simulink model "S_land_interfer_simulation"  (R2021a)
settings: Solver=FixedStepAuto  StartTime=0.0  StopTime=5  FixedStep=0.001  RelTol=1e-3
InitFcn:
  | Init_control;
values from neighbouring files (symbols this model uses):
  DEG2RAD = 0.0174533    [Init_control.m]
  Kd_PITCH_AgngleRate = 0.001    [Init_control.m]
  Kd_ROLL_AgngleRate = 0.001    [Init_control.m]
  Kd_YAW_AngleRate = 0.00    (= 0)    [Init_control.m]
  Ki_PITCH_AgngleRate = 0.10    (= 0.1)    [Init_control.m]
  Ki_ROLL_AgngleRate = 0.02    [Init_control.m]
  Ki_YAW_AngleRate = 0.01    [Init_control.m]
  Kp_PITCH_AgngleRate = 0.1    [Init_control.m]
  Kp_PITCH_ANGLE = 6.5    [Init_control.m]
  Kp_ROLL_AgngleRate = 0.1    [Init_control.m]
  Kp_ROLL_ANGLE = 6.5    [Init_control.m]
  Kp_YAW_AngleRate = 0.3    [Init_control.m]
  Kpxd = 0.5    [Init_control.m]
  Kpxi = 0    [Init_control.m]
  Kpxp = 5    [Init_control.m]
  Kpyp = 1.0    (= 1)    [Init_control.m]
  Kpzd = 0    [Init_control.m]
  Kpzi = 0.1    [Init_control.m]
  Kpzp = 5    [Init_control.m]
  Kvxd = 0.5    [Init_control.m]
  Kvxi = 0.01    [Init_control.m]
  Kvxp = 5    [Init_control.m]
  Kvyd = 0.01    [Init_control.m]
  Kvyi = 0    [Init_control.m]
  Kvyp = 2.0    (= 2)    [Init_control.m]
  Kvzd = 0.005    [Init_control.m]
  Kvzi = 0.01    [Init_control.m]
  Kvzp = 5    [Init_control.m]
  MAX_CONTROL_ANGLE_PITCH = 50    [Init_control.m]
  MAX_CONTROL_ANGLE_RATE_PITCH = 220    [Init_control.m]
  MAX_CONTROL_ANGLE_RATE_ROLL = 220    [Init_control.m]
  MAX_CONTROL_ANGLE_ROLL = 35    [Init_control.m]
  MAX_CONTROL_VELOCITY_XY = 5    [Init_control.m]
  MAX_CONTROL_VELOCITY_Z = 3    [Init_control.m]
  MAX_MAN_THR = 0.9    [Init_control.m]
  ModelInit_PosE = [0,0,-10]    [Init_control.m]
  ModelInit_RPM = 557.1420    (= 557.142)    [Init_control.m]
  RAD2DEG = 57.2957795    [Init_control.m]
  Saturation_I_ah = 3.431    [Init_control.m]
  Saturation_I_az = 5    [Init_control.m]
  Saturation_I_RP_Max = 0.3    [Init_control.m]
  Saturation_I_RP_Min = -0.3    [Init_control.m]
  Saturation_I_Y_Max = 0.2    [Init_control.m]
  Saturation_I_Y_Min = -0.2    [Init_control.m]
  THR_HOVER = 0.609    [Init_control.m]
undefined symbols (not defined in the file or in its folder): DiscIntNeverNeededParam, ModelParam_envGravityAcc, ModelParam_motorCr, ModelParam_motorJm, ModelParam_motorT, ModelParam_motorWb, ModelParam_rotorCm, ModelParam_rotorCt, ModelParam_uavCd, ModelParam_uavJ, ModelParam_uavMass, ModelParam_uavR
libraries: simulink x5, sharedutil x2, pid_lib x2, sharedtransform x1
settings Model: Creator=dream  LastModifiedBy=shenl
settings SolverCC: AlgebraicLoopSolver=TrustRegion
settings DataIOCC: ReturnWorkspaceOutputs=off
settings DebuggingCC: BusObjectLabelMismatch=error  SFMachineParentedDataDiag=warning  ArithmeticOperatorsInVariantConditions=warning
settings SFSimCC: SimUseLocalCustomCode=off  CustomCodeUndefinedFunction=UseInterfaceOnly
settings RTWCC: RTWUseLocalCustomCode=off
settings CodeAppCC: StateflowObjectComments=on

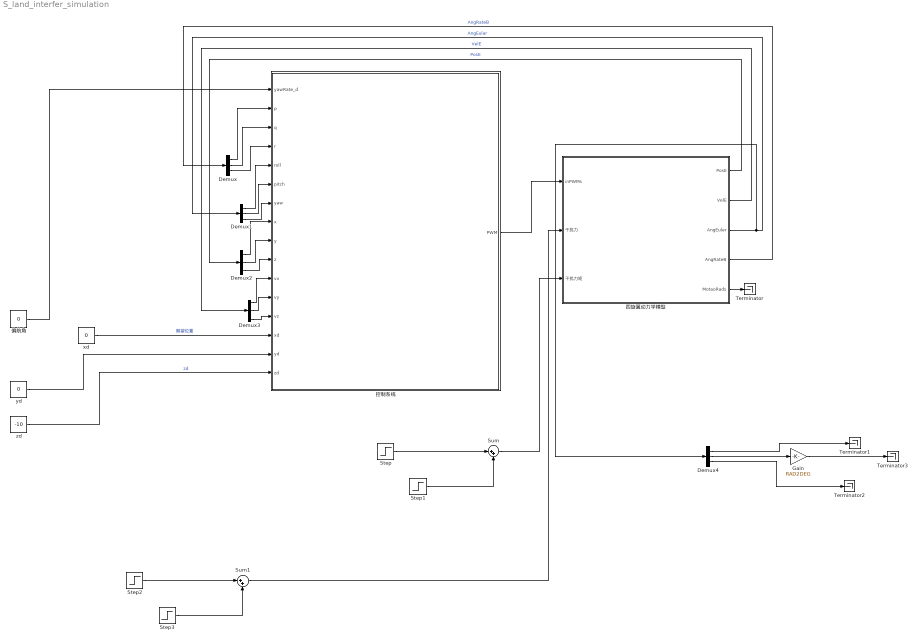
== system S_land_interfer_simulation ==
  Demux{,1..4} (5 alike) : Demux  Outputs=3
  Gain : Gain  Gain=RAD2DEG
  Step : Step  After=7  SampleTime=0
  Step1 : Step  Time=1.1  After=-6.1  SampleTime=0
  Step2 : Step  After=36  SampleTime=0
  Step3 : Step  Time=1.1  After=-30  SampleTime=0
  Sum : Sum  Inputs=|++
  Sum1 : Sum  Inputs=|++
  Terminator{,1..3} (4 alike) : Terminator
  xd : Constant  Value=0
  yd : Constant  Value=0
  zd : Constant  Value=-10
  偏航角 : Constant  Value=0  OutDataTypeStr=double
  "四旋翼动力学模型 " : Subsystem
      mask Display: image('./icon/F450.png');
  控制系统 : Subsystem
      mask Display: image('icon\pixhawk.png');
  wires:
  "四旋翼动力学模型 "/1(PosE) -> Demux2/1  "PosE"
  "四旋翼动力学模型 "/3(AngEuler) -> Demux4/1, Demux1/1  "AngEular"
  "四旋翼动力学模型 "/4(AngRateB) -> Demux/1  "AngRateB"
  Demux/1 -> 控制系统/2(p)
  Demux/2 -> 控制系统/3(q)
  Demux/3 -> 控制系统/4(r)
  Demux1/1 -> 控制系统/5(roll)
  Demux1/2 -> 控制系统/6(pitch)
  Demux1/3 -> 控制系统/7(yaw)
  Demux2/1 -> 控制系统/8(x)
  Demux2/2 -> 控制系统/9(y)
  Demux2/3 -> 控制系统/10(z)
  Demux3/1 -> 控制系统/11(vx)
  Demux3/2 -> 控制系统/12(vy)
  Demux3/3 -> 控制系统/13(vz)
  "四旋翼动力学模型 "/2(VelE) -> Demux3/1  "VelE"
  偏航角/1 -> 控制系统/1(yawRate_d)
  控制系统/1(PWM) -> "四旋翼动力学模型 "/1(inPWMs)
  "四旋翼动力学模型 "/5(MotaoRads) -> Terminator/1
  yd/1 -> 控制系统/15(yd)
  zd/1 -> 控制系统/16(zd)  "zd"
  Step/1 -> Sum/1
  Step1/1 -> Sum/2
  Sum/1 -> "四旋翼动力学模型 "/3(干扰力矩)
  Demux4/2 -> Gain/1
  Demux4/1 -> Terminator1/1
  Demux4/3 -> Terminator2/1
  Gain/1 -> Terminator3/1
  xd/1 -> 控制系统/14(xd)  "期望位置"
  Sum1/1 -> "四旋翼动力学模型 "/2(干扰力)
  Step3/1 -> Sum1/2
  Step2/1 -> Sum1/1

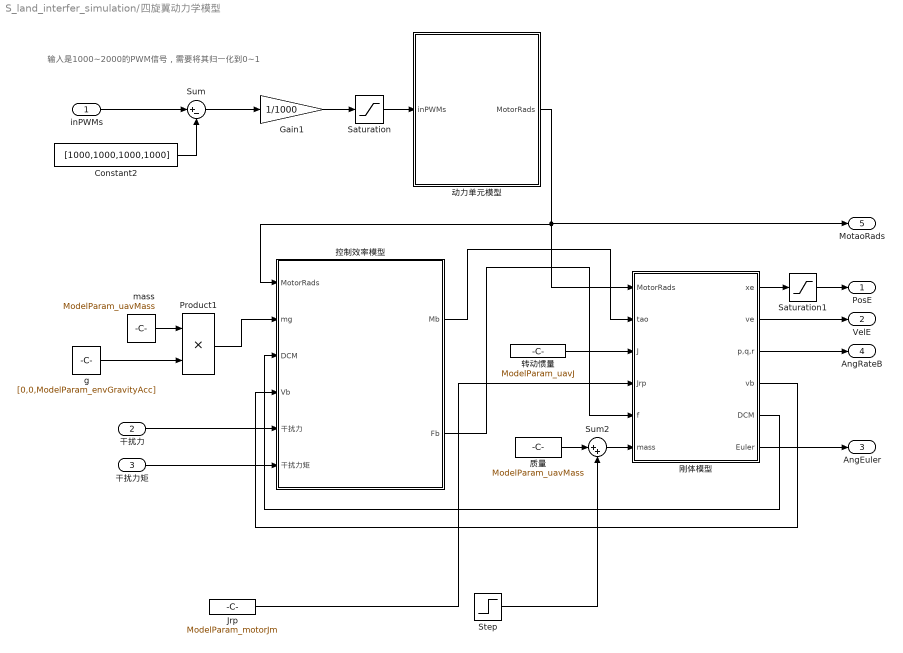
== system S_land_interfer_simulation/四旋翼动力学模型  ==
  note: 输入是1000~2000的PWM信号，需要将其归一化到0~1
  inPWMs : Inport
  干扰力 : Inport  Port=2
  干扰力矩 : Inport  Port=3
  Constant2 : Constant  Value=[1000,1000,1000,1000]
  Gain1 : Gain  Gain=1/1000
  Jrp : Constant  Value=ModelParam_motorJm
  Product1 : Product
  Saturation : Saturate  UpperLimit=1  LowerLimit=0
  Saturation1 : Saturate  UpperLimit=[inf,inf,0]  LowerLimit=[-inf,-inf,-inf]
  Step : Step  SampleTime=0
  Sum : Sum  Inputs=|+-
  Sum2 : Sum  Inputs=|++
  g : Constant  Value=[0,0,ModelParam_envGravityAcc]
  mass : Constant  Value=ModelParam_uavMass
  刚体模型 : Subsystem
  动力单元模型 : Subsystem
  控制效率模型 : Subsystem
  质量 : Constant  Value=ModelParam_uavMass
  转动惯量 : Constant  Value=ModelParam_uavJ
  PosE : Outport
  VelE : Outport  Port=2
  AngEuler : Outport  Port=3
  AngRateB : Outport  Port=4
  MotaoRads : Outport  Port=5
  wires:
  Saturation/1 -> 动力单元模型/1(inPWMs)
  刚体模型/3("p,q,r ") -> AngRateB/1
  质量/1 -> Sum2/1
  刚体模型/5(DCM) -> 控制效率模型/3(DCM)
  刚体模型/1("xe ") -> Saturation1/1
  动力单元模型/1(MotorRads) -> 控制效率模型/1(MotorRads), 刚体模型/1(MotorRads), MotaoRads/1
  转动惯量/1 -> 刚体模型/3(J)
  Gain1/1 -> Saturation/1
  刚体模型/2(ve) -> VelE/1
  Sum/1 -> Gain1/1
  Product1/1 -> 控制效率模型/2(mg)
  刚体模型/4("vb ") -> 控制效率模型/4(Vb)
  Saturation1/1 -> PosE/1
  刚体模型/6(Euler) -> AngEuler/1
  控制效率模型/1(Mb) -> 刚体模型/2(tao)
  inPWMs/1 -> Sum/1
  控制效率模型/2(Fb) -> 刚体模型/5(f)
  Constant2/1 -> Sum/2
  g/1 -> Product1/2
  干扰力/1 -> 控制效率模型/5(干扰力)
  mass/1 -> Product1/1
  干扰力矩/1 -> 控制效率模型/6(干扰力矩)
  Sum2/1 -> 刚体模型/6(mass)
  Step/1 -> Sum2/2
  Jrp/1 -> 刚体模型/4(Jrp)

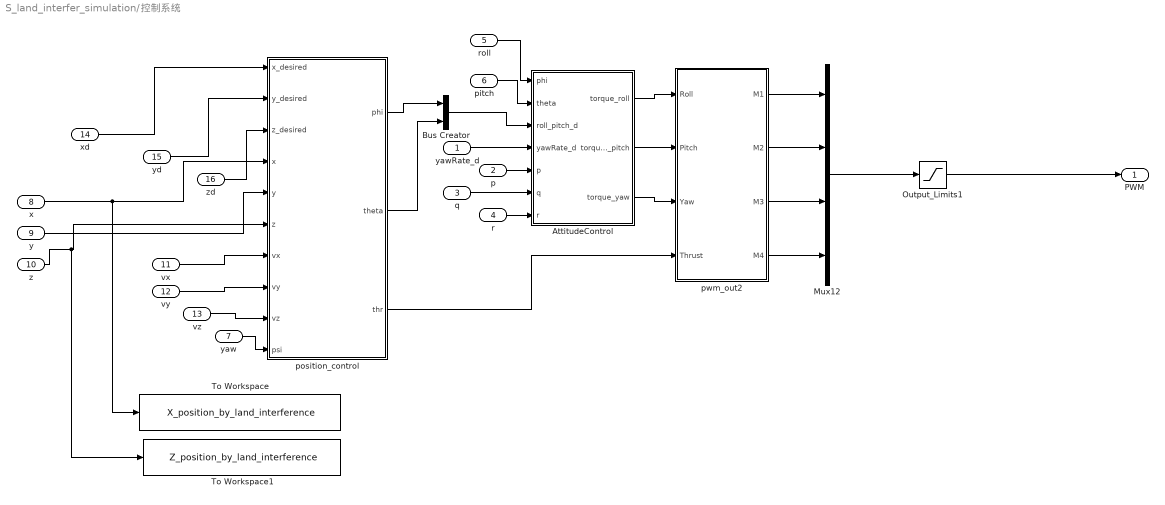
== system S_land_interfer_simulation/控制系统 ==
  yawRate_d : Inport
  p : Inport  Port=2  PortDimensions=1
  q : Inport  Port=3  PortDimensions=1
  r : Inport  Port=4  PortDimensions=1
  roll : Inport  Port=5  PortDimensions=1
  pitch : Inport  Port=6  PortDimensions=1
  yaw : Inport  Port=7  PortDimensions=1
  x : Inport  Port=8
  y : Inport  Port=9
  z : Inport  Port=10
  vx : Inport  Port=11
  vy : Inport  Port=12
  vz : Inport  Port=13
  xd : Inport  Port=14
  yd : Inport  Port=15
  zd : Inport  Port=16
  AttitudeControl : Subsystem
  Bus Creator : BusCreator  Inputs=2
  Mux12 : Mux
  Output_Limits1 : Saturate  UpperLimit=2000  LowerLimit=1000
  To Workspace : ToWorkspace  VariableName=X_position_by_land_interference  SaveFormat=Timeseries  SampleTime=-1
  To Workspace1 : ToWorkspace  VariableName=Z_position_by_land_interference  SaveFormat=Timeseries  SampleTime=-1
  position_control : Subsystem
  pwm_out2 : MATLAB Function  SystemSampleTime=0.004
  PWM : Outport  PortDimensions=4
  wires:
  Mux12/1 -> Output_Limits1/1
  AttitudeControl/2(torque_pitch) -> pwm_out2/2(Pitch)
  AttitudeControl/1(torque_roll) -> pwm_out2/1(Roll)
  pwm_out2/1(M1) -> Mux12/1
  pwm_out2/3(M3) -> Mux12/3
  pwm_out2/2(M2) -> Mux12/2
  AttitudeControl/3(torque_yaw) -> pwm_out2/3(Yaw)
  yawRate_d/1 -> AttitudeControl/4(yawRate_d)
  p/1 -> AttitudeControl/5(p)
  pwm_out2/4(M4) -> Mux12/4
  roll/1 -> AttitudeControl/1(phi)
  pitch/1 -> AttitudeControl/2(theta)
  position_control/1(phi) -> Bus Creator/1
  position_control/2(theta) -> Bus Creator/2
  Bus Creator/1 -> AttitudeControl/3(roll_pitch_d)
  position_control/3(thr) -> pwm_out2/4(Thrust)
  x/1 -> To Workspace/1, position_control/4(x)
  y/1 -> position_control/5(y)
  z/1 -> To Workspace1/1, position_control/6(z)
  vx/1 -> position_control/7(vx)
  vy/1 -> position_control/8(vy)
  vz/1 -> position_control/9(vz)
  yaw/1 -> position_control/10(psi)
  Output_Limits1/1 -> PWM/1
  r/1 -> AttitudeControl/7(r)
  q/1 -> AttitudeControl/6(q)
  xd/1 -> position_control/1(x_desired)
  yd/1 -> position_control/2(y_desired)
  zd/1 -> position_control/3(z_desired)

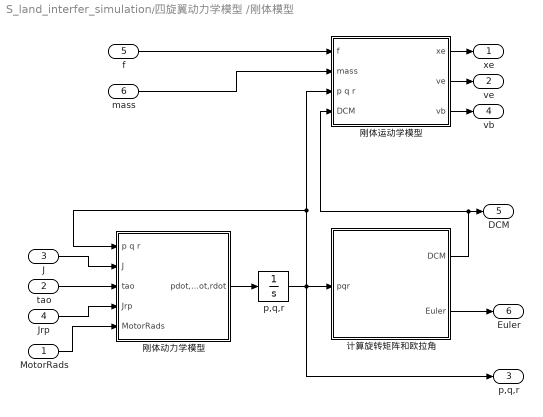
== system S_land_interfer_simulation/四旋翼动力学模型 /刚体模型 ==
  MotorRads : Inport
  tao : Inport  Port=2
  J : Inport  Port=3
  Jrp : Inport  Port=4
  f : Inport  Port=5
  mass : Inport  Port=6
  p,q,r : Integrator
  刚体动力学模型 : Subsystem
  刚体运动学模型 : Subsystem
  计算旋转矩阵和欧拉角 : Subsystem
  "xe " : Outport
  ve : Outport  Port=2
  "p,q,r " : Outport  Port=3
  "vb " : Outport  Port=4
  DCM : Outport  Port=5
  Euler : Outport  Port=6
  wires:
  刚体运动学模型/3("vb ") -> "vb "/1
  p,q,r/1 -> 计算旋转矩阵和欧拉角/1(pqr), "p,q,r "/1, 刚体动力学模型/1(p q r), 刚体运动学模型/3(p q r)
  刚体运动学模型/2(ve) -> ve/1
  刚体运动学模型/1("xe ") -> "xe "/1
  mass/1 -> 刚体运动学模型/2(mass)
  f/1 -> 刚体运动学模型/1(f)
  计算旋转矩阵和欧拉角/2(Euler) -> Euler/1
  计算旋转矩阵和欧拉角/1(DCM) -> 刚体运动学模型/4(DCM), DCM/1
  刚体动力学模型/1(pdot,qdot,rdot) -> p,q,r/1
  MotorRads/1 -> 刚体动力学模型/5(MotorRads)
  Jrp/1 -> 刚体动力学模型/4(Jrp)
  tao/1 -> 刚体动力学模型/3(tao)
  J/1 -> 刚体动力学模型/2(J)

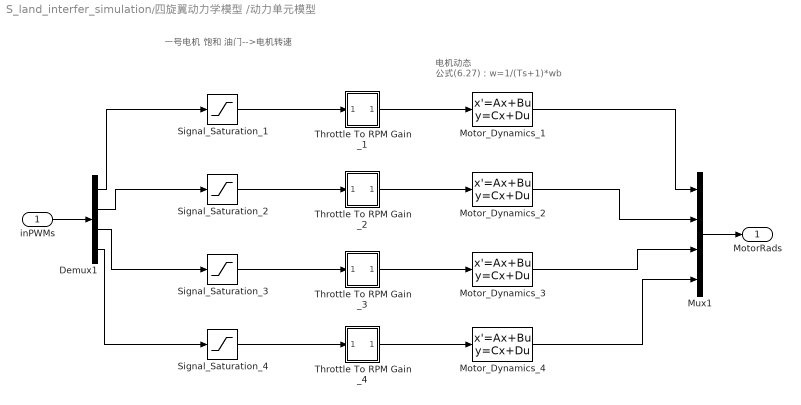
== system S_land_interfer_simulation/四旋翼动力学模型 /动力单元模型 ==
  note: 电机动态
      | 公式(6.27)：w=1/(Ts+1)*wb
  note: 一号电机
      |
      |              饱和                             油门-->电机转速
  inPWMs : Inport
  Demux1 : Demux
  Motor_Dynamics_{1..4} (4 alike) : StateSpace  A=-1/ModelParam_motorT  C=1/ModelParam_motorT  D=0  InitialCondition=ModelInit_RPM*ModelParam_motorT
  Mux1 : Mux
  Signal_Saturation_{1..4} (4 alike) : Saturate  UpperLimit=1  LowerLimit=0
  Throttle To RPM Gain _1 : Subsystem
  Throttle To RPM Gain _2 : Subsystem
  Throttle To RPM Gain _3 : Subsystem
  Throttle To RPM Gain _4 : Subsystem
  MotorRads : Outport
  wires:
  Throttle To RPM Gain _4/1(Out5) -> Motor_Dynamics_4/1
  Signal_Saturation_4/1 -> Throttle To RPM Gain _4/1(In5)
  Signal_Saturation_3/1 -> Throttle To RPM Gain _3/1(In5)
  Signal_Saturation_2/1 -> Throttle To RPM Gain _2/1(In5)
  Motor_Dynamics_4/1 -> Mux1/4
  Motor_Dynamics_3/1 -> Mux1/3
  Motor_Dynamics_2/1 -> Mux1/2
  Motor_Dynamics_1/1 -> Mux1/1
  Signal_Saturation_1/1 -> Throttle To RPM Gain _1/1(In5)
  Mux1/1 -> MotorRads/1
  Throttle To RPM Gain _3/1(Out5) -> Motor_Dynamics_3/1
  Throttle To RPM Gain _2/1(Out5) -> Motor_Dynamics_2/1
  Throttle To RPM Gain _1/1(Out5) -> Motor_Dynamics_1/1
  inPWMs/1 -> Demux1/1
  Demux1/4 -> Signal_Saturation_4/1
  Demux1/3 -> Signal_Saturation_3/1
  Demux1/2 -> Signal_Saturation_2/1
  Demux1/1 -> Signal_Saturation_1/1

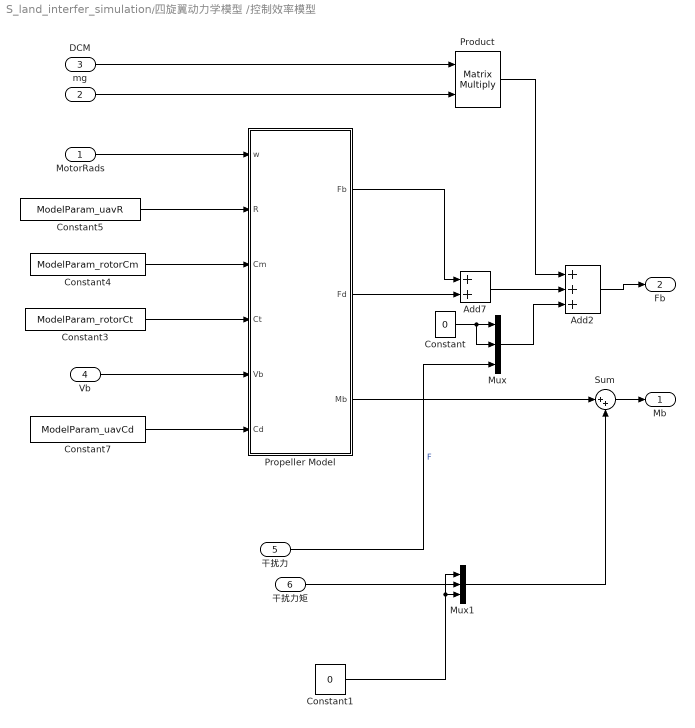
== system S_land_interfer_simulation/四旋翼动力学模型 /控制效率模型 ==
  MotorRads : Inport
  mg : Inport  Port=2
  DCM : Inport  Port=3
  Vb : Inport  Port=4
  干扰力 : Inport  Port=5
  干扰力矩 : Inport  Port=6
  Add2 : Sum  Inputs=+++
  Add7 : Sum
  Constant : Constant  Value=0
  Constant1 : Constant  Value=0
  Constant3 : Constant  Value=ModelParam_rotorCt
  Constant4 : Constant  Value=ModelParam_rotorCm
  Constant5 : Constant  Value=ModelParam_uavR
  Constant7 : Constant  Value=ModelParam_uavCd
  Mux : Mux  Inputs=3
  Mux1 : Mux  Inputs=3
  Product : Product  Multiplication=Matrix(*)
  Propeller Model : MATLAB Function  TreatAsAtomicUnit=on
  Sum : Sum  Inputs=|++
  Mb : Outport
  Fb : Outport  Port=2
  wires:
  Propeller Model/3(Mb) -> Sum/1
  Add2/1 -> Fb/1
  Constant3/1 -> Propeller Model/4(Ct)
  Propeller Model/2(Fd) -> Add7/2
  Add7/1 -> Add2/2
  Propeller Model/1(Fb) -> Add7/1
  Product/1 -> Add2/1
  mg/1 -> Product/2
  DCM/1 -> Product/1
  Constant7/1 -> Propeller Model/6(Cd)
  Vb/1 -> Propeller Model/5(Vb)
  Constant5/1 -> Propeller Model/2(R)
  Constant4/1 -> Propeller Model/3(Cm)
  MotorRads/1 -> Propeller Model/1(w)
  Constant/1 -> Mux/2, Mux/1
  干扰力/1 -> Mux/3  "F"
  Mux/1 -> Add2/3
  Sum/1 -> Mb/1
  Mux1/1 -> Sum/2
  干扰力矩/1 -> Mux1/2
  Constant1/1 -> Mux1/1, Mux1/3

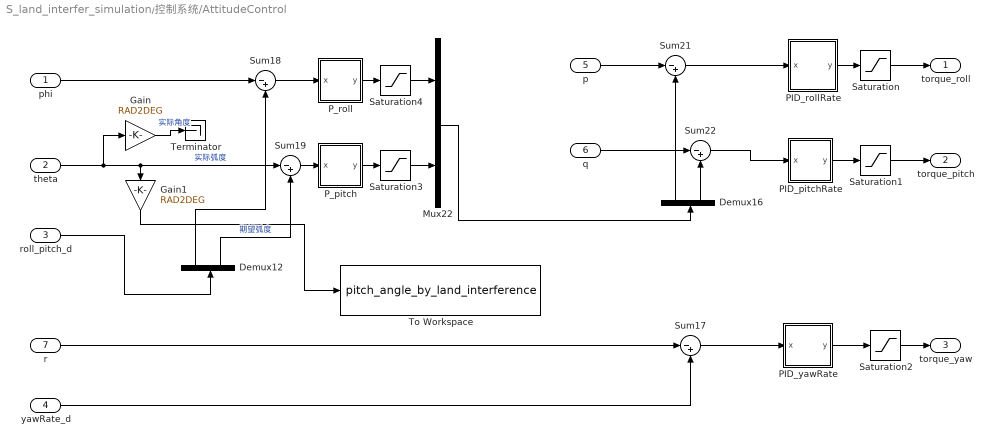
== system S_land_interfer_simulation/控制系统/AttitudeControl ==
  phi : Inport
  theta : Inport  Port=2
  roll_pitch_d : Inport  Port=3
  yawRate_d : Inport  Port=4
  p : Inport  Port=5
  q : Inport  Port=6
  r : Inport  Port=7
  Demux12 : Demux  Outputs=2
  Demux16 : Demux  Outputs=2
  Gain : Gain  Gain=RAD2DEG
  Gain1 : Gain  Gain=RAD2DEG
  Mux22 : Mux  Inputs=2
  PID_pitchRate : Subsystem
  PID_rollRate : Subsystem
  PID_yawRate : Subsystem
  "P_pitch " : Subsystem
  "P_roll " : Subsystem
  Saturation : Saturate  UpperLimit=1  LowerLimit=-1
  Saturation1 : Saturate  UpperLimit=1  LowerLimit=-1
  Saturation2 : Saturate
  Saturation3 : Saturate  UpperLimit=MAX_CONTROL_ANGLE_RATE_PITCH  LowerLimit=-MAX_CONTROL_ANGLE_RATE_PITCH
  Saturation4 : Saturate  UpperLimit=MAX_CONTROL_ANGLE_RATE_ROLL  LowerLimit=-MAX_CONTROL_ANGLE_RATE_ROLL
  Sum{17..19,21..22} (5 alike) : Sum  Inputs=|-+
  Terminator : Terminator
  To Workspace : ToWorkspace  VariableName=pitch_angle_by_land_interference  SaveFormat=Timeseries  SampleTime=-1
  torque_roll : Outport
  torque_pitch : Outport  Port=2
  torque_yaw : Outport  Port=3
  wires:
  r/1 -> Sum17/1
  Sum19/1 -> "P_pitch "/1(x)
  "P_pitch "/1(y) -> Saturation3/1
  "P_roll "/1(y) -> Saturation4/1
  roll_pitch_d/1 -> Demux12/1
  Demux12/1 -> Sum18/2
  phi/1 -> Sum18/1
  theta/1 -> Gain/1, Gain1/1, Sum19/1  "实际弧度"
  Sum18/1 -> "P_roll "/1(x)
  Sum22/1 -> PID_pitchRate/1(x)
  Sum17/1 -> PID_yawRate/1(x)
  p/1 -> Sum21/1
  q/1 -> Sum22/1
  Sum21/1 -> PID_rollRate/1(x)
  Demux16/1 -> Sum21/2
  PID_pitchRate/1(y) -> Saturation1/1
  PID_rollRate/1(y) -> Saturation/1
  PID_yawRate/1(y) -> Saturation2/1
  yawRate_d/1 -> Sum17/2
  Saturation/1 -> torque_roll/1
  Saturation1/1 -> torque_pitch/1
  Saturation2/1 -> torque_yaw/1
  Mux22/1 -> Demux16/1
  Saturation4/1 -> Mux22/1
  Saturation3/1 -> Mux22/2
  Demux16/2 -> Sum22/2
  Demux12/2 -> Sum19/2  "期望弧度"
  Gain/1 -> Terminator/1  "实际角度"
  Gain1/1 -> To Workspace/1

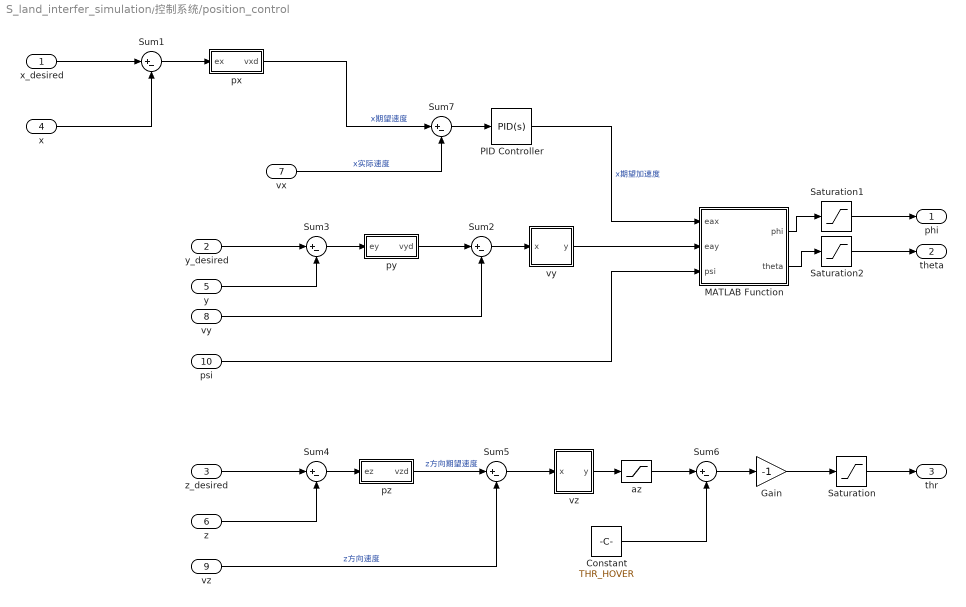
== system S_land_interfer_simulation/控制系统/position_control ==
  x_desired : Inport
  y_desired : Inport  Port=2
  z_desired : Inport  Port=3  OutDataTypeStr=double
  x : Inport  Port=4
  y : Inport  Port=5
  z : Inport  Port=6  OutDataTypeStr=double
  vx : Inport  Port=7
  vy : Inport  Port=8
  vz : Inport  Port=9  OutDataTypeStr=double
  psi : Inport  Port=10
  Constant : Constant  Value=THR_HOVER
  Gain : Gain  Gain=-1
  MATLAB Function : MATLAB Function  TreatAsAtomicUnit=on
  PID Controller : pid_lib/PID Controller  Controller=PID  Form=Parallel  TimeDomain=Continuous-time  UseExternalTs=off  SampleTime=-1  IntegratorMethod=Forward Euler  FilterMethod=Forward Euler  ControllerParametersSource=internal  P=Kvxp  I=Kvxi  D=Kvxd  UseFilter=on  N=100  TunerSelectOption=Transfer Function Based (PID Tuner App)  InitialConditionSource=internal  InitialConditionForIntegrator=0  InitialConditionForFilter=0  DifferentiatorICPrevScaledInput=0  ExternalReset=none  TrackingMode=off  Kt=1  LimitOutput=off  SatLimitsSource=internal  UpperSaturationLimit=inf  LowerSaturationLimit=-inf  LinearizeAsGain=on  AntiWindupMode=none  Kb=1  POutMin=[]  POutMax=[]  IOutMin=[]  IOutMax=[]  DOutMin=[]  DOutMax=[]  NOutMin=[]  NOutMax=[]  SumOutMin=[]  SumOutMax=[]  SaturationOutMin=[]  SaturationOutMax=[]  PParamMin=[]  PParamMax=[]  IParamMin=[]  IParamMax=[]  DParamMin=[]  DParamMax=[]  NParamMin=[]  NParamMax=[]  KbParamMin=[]  KbParamMax=[]  KtParamMin=[]  KtParamMax=[]  KbOutMin=[]  KbOutMax=[]  KtOutMin=[]  KtOutMax=[]  IntegratorOutMin=[]  IntegratorOutMax=[]  FilterOutMin=[]  FilterOutMax=[]  SumI1OutMin=[]  SumI1OutMax=[]  SumI2OutMin=[]  SumI2OutMax=[]  SumI3OutMin=[]  SumI3OutMax=[]  SumI4OutMin=[]  SumI4OutMax=[]  SumDOutMin=[]  SumDOutMax=[]  DifferentiatorOutMin=[]  DifferentiatorOutMax=[]  FilterDiffOutCoefMin=[]  FilterDiffOutCoefMax=[]  ReciprocalOutMin=[]  ReciprocalOutMax=[]  SumDenOutMin=[]  SumDenOutMax=[]  SumNumOutMin=[]  SumNumOutMax=[]  DivideOutMin=[]  DivideOutMax=[]  UdiffTsProdOutMin=[]  UdiffTsProdOutMax=[]  NTsProdOutMin=[]  NTsProdOutMax=[]  UintegralTsProdOutMin=[]  UintegralTsProdOutMax=[]  UngainTsProdOutMin=[]  UngainTsProdOutMax=[]  IntegratorContinuousStateAttributes=''  IntegratorStateMustResolveToSignalObject=off  IntegratorRTWStateStorageClass=Auto  FilterContinuousStateAttributes=''  FilterStateMustResolveToSignalObject=off  FilterRTWStateStorageClass=Auto  ParallelPVariant=InternalParameters  IdealPVariant=Disabled  IVariant=InternalParameters  DVariant=InternalParameters  IntegratorVariant=Continuous  SatVariant=Disabled  AWVariant=Passthrough  PCopyVariant=Disabled  TRVariant=Disabled  FdbkBlocksVariant=Forward  IdealPFdbkVariant=Disabled  SatFdbkVariant=Disabled  DerivativeFilterVariant=ContFilter  NVariant=InternalParameters  NCopyVariant=Disabled  FilterICVariant=InternalICsFilter  IntegratorICVariant=InternalICs  ExternalResetVariant=Disabled  TRSumVariant=Passthrough  SumFdbkVariant=Disabled  SumVariant=Sum_PID  TsampFilterVariant=InternalTs  TsampNgainVariant=Passthrough  TsampIntegralVariant=Passthrough  ExternalSaturationOutDataTypeStr=Inherit: Same as second input
  Saturation : Saturate  UpperLimit=MAX_MAN_THR  LowerLimit=0
  Saturation1 : Saturate  UpperLimit=MAX_CONTROL_ANGLE_ROLL*DEG2RAD  LowerLimit=-MAX_CONTROL_ANGLE_ROLL*DEG2RAD
  Saturation2 : Saturate  UpperLimit=MAX_CONTROL_ANGLE_PITCH*DEG2RAD  LowerLimit=-MAX_CONTROL_ANGLE_PITCH*DEG2RAD
  Sum{1..7} (7 alike) : Sum  Inputs=|+-
  az : Saturate  UpperLimit=0.4  LowerLimit=-0.4
  px : Subsystem
  py : Subsystem
  pz : Subsystem
  "vy " : Subsystem
  "vz " : Subsystem
  phi : Outport
  theta : Outport  Port=2
  thr : Outport  Port=3
  wires:
  Saturation/1 -> thr/1
  Gain/1 -> Saturation/1
  Sum6/1 -> Gain/1
  "vz "/1(y) -> az/1
  Sum4/1 -> pz/1(ez)
  z/1 -> Sum4/2
  Constant/1 -> Sum6/2
  Sum5/1 -> "vz "/1(x)
  vz/1 -> Sum5/2  "z方向速度"
  x/1 -> Sum1/2
  y/1 -> Sum3/2
  Sum3/1 -> py/1(ey)
  y_desired/1 -> Sum3/1
  vy/1 -> Sum2/2
  Sum2/1 -> "vy "/1(x)
  Sum7/1 -> PID Controller/1
  Sum1/1 -> px/1(ex)
  pz/1(vzd) -> Sum5/1  "z方向期望速度"
  z_desired/1 -> Sum4/1
  Saturation1/1 -> phi/1
  Saturation2/1 -> theta/1
  psi/1 -> MATLAB Function/3(psi)
  py/1(vyd) -> Sum2/1
  MATLAB Function/1(phi) -> Saturation1/1
  MATLAB Function/2(theta) -> Saturation2/1
  "vy "/1(y) -> MATLAB Function/2(eay)
  az/1 -> Sum6/1
  vx/1 -> Sum7/2  "x实际速度"
  x_desired/1 -> Sum1/1
  px/1(vxd) -> Sum7/1  "x期望速度"
  PID Controller/1 -> MATLAB Function/1(eax)  "x期望加速度"

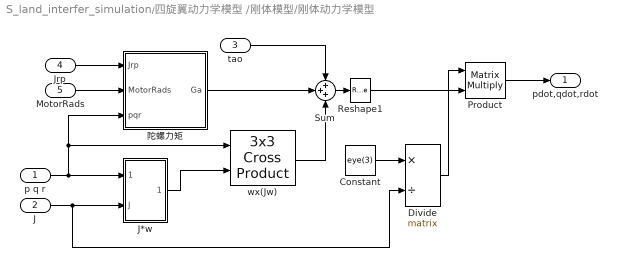
== system S_land_interfer_simulation/四旋翼动力学模型 /刚体模型/刚体动力学模型 ==
  p q r : Inport
  J : Inport  Port=2
  tao : Inport  Port=3
  Jrp : Inport  Port=4
  MotorRads : Inport  Port=5
  Constant : Constant  Value=eye(3)
  Divide : Product  Inputs=*/  Multiplication=Matrix(*)
  J*w : Subsystem
  Product : Product  Multiplication=Matrix(*)
  Reshape1 : Reshape  OutputDimensionality=Column vector (2-D)
  Sum : Sum  Inputs=3
  wx(Jw) : sharedutil/3x3 Cross Product  aMode=aMode
      settings: SourceProductBaseCode=AE,PW,DR,MT,UV,VE
  陀螺力矩 : MATLAB Function  TreatAsAtomicUnit=on
  pdot,qdot,rdot : Outport
  wires:
  Product/1 -> pdot,qdot,rdot/1
  Reshape1/1 -> Product/2
  Constant/1 -> Divide/1
  陀螺力矩/1(Ga) -> Sum/2
  Divide/1 -> Product/1
  Sum/1 -> Reshape1/1
  J/1 -> Divide/2, J*w/2(J)
  p q r/1 -> J*w/1(p q r), 陀螺力矩/3(pqr), wx(Jw)/1
  J*w/1("J*w ") -> wx(Jw)/2
  tao/1 -> Sum/1
  Jrp/1 -> 陀螺力矩/1(Jrp)
  MotorRads/1 -> 陀螺力矩/2(MotorRads)
  wx(Jw)/1 -> Sum/3

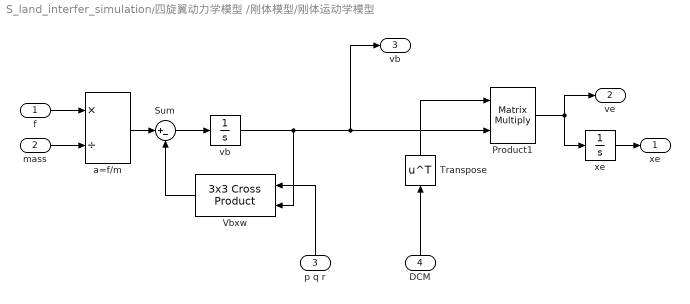
== system S_land_interfer_simulation/四旋翼动力学模型 /刚体模型/刚体运动学模型 ==
  f : Inport
  mass : Inport  Port=2
  p q r : Inport  Port=3
  DCM : Inport  Port=4
  Product1 : Product  Multiplication=Matrix(*)
  Sum : Sum  Inputs=|+-
  Transpose : Math  Operator=transpose  SignedPower=on  SaturateOnIntegerOverflow=on
  Vbxw : sharedutil/3x3 Cross Product  aMode=aMode
      settings: SourceProductBaseCode=AE,PW,DR,MT,UV,VE
  a=f/m : Product  Inputs=*/
  vb : Integrator
  xe : Integrator  InitialCondition=ModelInit_PosE
  "xe " : Outport
  ve : Outport  Port=2
  "vb " : Outport  Port=3
  wires:
  vb/1 -> Product1/2, "vb "/1, Vbxw/2
  a=f/m/1 -> Sum/1
  Sum/1 -> vb/1
  xe/1 -> "xe "/1
  Product1/1 -> xe/1, ve/1
  Transpose/1 -> Product1/1
  mass/1 -> a=f/m/2
  Vbxw/1 -> Sum/2
  f/1 -> a=f/m/1
  p q r/1 -> Vbxw/1
  DCM/1 -> Transpose/1

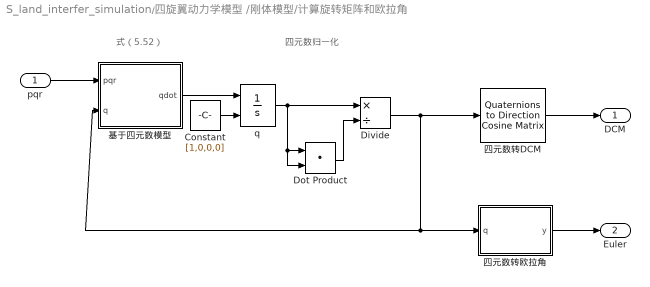
== system S_land_interfer_simulation/四旋翼动力学模型 /刚体模型/计算旋转矩阵和欧拉角 ==
  note: 式（5.52）
  note: 四元数归一化
  pqr : Inport
  Constant : Constant  Value=[1,0,0,0]
  Divide : Product  Inputs=*/
  Dot Product : DotProduct  InputSameDT=on  OutDataTypeStr=Inherit: Inherit via internal rule
  q : Integrator  InitialConditionSource=external
  四元数转DCM : sharedtransform/Quaternions to  Direction Cosine Matrix  aMode=aMode
      settings: SourceProductBaseCode=AE,PW,DR,MT,UV,VE
  四元数转欧拉角 : MATLAB Function
  基于四元数模型 : MATLAB Function  TreatAsAtomicUnit=on
  DCM : Outport
  Euler : Outport  Port=2
  wires:
  四元数转欧拉角/1(y) -> Euler/1
  Divide/1 -> 四元数转DCM/1, 基于四元数模型/2(q), 四元数转欧拉角/1(q)
  Dot Product/1 -> Divide/2
  四元数转DCM/1 -> DCM/1
  pqr/1 -> 基于四元数模型/1(pqr)
  q/1 -> Dot Product/1, Dot Product/2, Divide/1
  基于四元数模型/1(qdot) -> q/1
  Constant/1 -> q/2

== system S_land_interfer_simulation/四旋翼动力学模型 /动力单元模型/Throttle To RPM Gain _1 ==
  In5 : Inport
  Constant : Constant  Value=ModelParam_motorWb
  Gain : Gain  Gain=ModelParam_motorCr
  Sum1 : Sum  Inputs=++|
  Out5 : Outport
  wires:
  Constant/1 -> Sum1/1
  Gain/1 -> Sum1/2
  In5/1 -> Gain/1
  Sum1/1 -> Out5/1

== system S_land_interfer_simulation/四旋翼动力学模型 /动力单元模型/Throttle To RPM Gain _2 ==
  In5 : Inport
  Constant : Constant  Value=ModelParam_motorWb
  Gain : Gain  Gain=ModelParam_motorCr
  Sum1 : Sum  Inputs=++|
  Out5 : Outport
  wires:
  Sum1/1 -> Out5/1
  In5/1 -> Gain/1
  Gain/1 -> Sum1/2
  Constant/1 -> Sum1/1

== system S_land_interfer_simulation/四旋翼动力学模型 /动力单元模型/Throttle To RPM Gain _3 ==
  In5 : Inport
  Constant : Constant  Value=ModelParam_motorWb
  Gain : Gain  Gain=ModelParam_motorCr
  Sum1 : Sum  Inputs=++|
  Out5 : Outport
  wires:
  Constant/1 -> Sum1/1
  Gain/1 -> Sum1/2
  In5/1 -> Gain/1
  Sum1/1 -> Out5/1

== system S_land_interfer_simulation/四旋翼动力学模型 /动力单元模型/Throttle To RPM Gain _4 ==
  In5 : Inport
  Constant : Constant  Value=ModelParam_motorWb
  Gain : Gain  Gain=ModelParam_motorCr
  Sum1 : Sum  Inputs=++|
  Out5 : Outport
  wires:
  Sum1/1 -> Out5/1
  In5/1 -> Gain/1
  Gain/1 -> Sum1/2
  Constant/1 -> Sum1/1

== system S_land_interfer_simulation/控制系统/AttitudeControl/PID_pitchRate ==
  x : Inport
  Derivative Gain : Gain  DisableCoverage=on  Gain=Kd_PITCH_AgngleRate  ParamMin=-100  ParamMax=100  OutMin=-100  OutMax=100
  Discrete Derivative : simulink/Discrete/Discrete Derivative  gainval=1.0  ICPrevScaledInput=0.0  OutMin=[]  OutMax=[]  OutDataType=fixdt(1, 16)  OutScaling=2^-10  DoSatur=off
  Discrete-Time Integrator : DiscreteIntegrator  SampleTime=-1  LimitOutput=on  UpperSaturationLimit=Saturation_I_RP_Max  LowerSaturationLimit=Saturation_I_RP_Min  ICPrevOutput=DiscIntNeverNeededParam  ICPrevScaledInput=DiscIntNeverNeededParam
  Gain : Gain  Gain=Kp_PITCH_AgngleRate
  Integral Gain : Gain  DisableCoverage=on  Gain=Ki_PITCH_AgngleRate
  Sum : Sum  Inputs=+++
  y : Outport  InitialOutput=0
  wires:
  Discrete-Time Integrator/1 -> Sum/2
  Discrete Derivative/1 -> Sum/3
  Sum/1 -> y/1
  Gain/1 -> Sum/1
  Derivative Gain/1 -> Discrete Derivative/1
  Integral Gain/1 -> Discrete-Time Integrator/1
  x/1 -> Derivative Gain/1, Integral Gain/1, Gain/1

== system S_land_interfer_simulation/控制系统/AttitudeControl/PID_rollRate ==
  x : Inport
  Derivative Gain : Gain  DisableCoverage=on  Gain=Kd_ROLL_AgngleRate  ParamMin=-100  ParamMax=100  OutMin=-100  OutMax=100
  Discrete Derivative : simulink/Discrete/Discrete Derivative  gainval=1.0  ICPrevScaledInput=0.0  OutMin=[]  OutMax=[]  OutDataType=fixdt(1, 16)  OutScaling=2^-10  DoSatur=off
  Discrete-Time Integrator : DiscreteIntegrator  SampleTime=-1  LimitOutput=on  UpperSaturationLimit=Saturation_I_RP_Max  LowerSaturationLimit=Saturation_I_RP_Min  ICPrevOutput=DiscIntNeverNeededParam  ICPrevScaledInput=DiscIntNeverNeededParam
  Gain : Gain  Gain=Kp_ROLL_AgngleRate
  Integral Gain : Gain  DisableCoverage=on  Gain=Ki_ROLL_AgngleRate
  Sum : Sum  Inputs=+++
  y : Outport  InitialOutput=0
  wires:
  x/1 -> Gain/1, Integral Gain/1, Derivative Gain/1
  Integral Gain/1 -> Discrete-Time Integrator/1
  Derivative Gain/1 -> Discrete Derivative/1
  Gain/1 -> Sum/1
  Sum/1 -> y/1
  Discrete Derivative/1 -> Sum/3
  Discrete-Time Integrator/1 -> Sum/2

== system S_land_interfer_simulation/控制系统/AttitudeControl/PID_yawRate ==
  x : Inport
  Derivative Gain : Gain  DisableCoverage=on  Gain=Kd_YAW_AngleRate  ParamMin=-100  ParamMax=100  OutMin=-100  OutMax=100
  Discrete Derivative : simulink/Discrete/Discrete Derivative  gainval=1.0  ICPrevScaledInput=0.0  OutMin=[]  OutMax=[]  OutDataType=fixdt(1, 16)  OutScaling=2^-10  DoSatur=off
  Discrete-Time Integrator : DiscreteIntegrator  SampleTime=-1  LimitOutput=on  UpperSaturationLimit=Saturation_I_Y_Max  LowerSaturationLimit=Saturation_I_Y_Min  ICPrevOutput=DiscIntNeverNeededParam  ICPrevScaledInput=DiscIntNeverNeededParam
  Gain : Gain  Gain=Kp_YAW_AngleRate
  Integral Gain : Gain  DisableCoverage=on  Gain=Ki_YAW_AngleRate
  Sum : Sum  Inputs=+++
  y : Outport  InitialOutput=0
  wires:
  x/1 -> Gain/1, Integral Gain/1, Derivative Gain/1
  Integral Gain/1 -> Discrete-Time Integrator/1
  Derivative Gain/1 -> Discrete Derivative/1
  Gain/1 -> Sum/1
  Sum/1 -> y/1
  Discrete Derivative/1 -> Sum/3
  Discrete-Time Integrator/1 -> Sum/2

== system S_land_interfer_simulation/控制系统/AttitudeControl/P_pitch  ==
  x : Inport
  Gain : Gain  Gain=Kp_PITCH_ANGLE
  y : Outport  InitialOutput=0
  wires:
  x/1 -> Gain/1
  Gain/1 -> y/1

== system S_land_interfer_simulation/控制系统/AttitudeControl/P_roll  ==
  x : Inport
  Gain : Gain  Gain=Kp_ROLL_ANGLE
  y : Outport  InitialOutput=0
  wires:
  Gain/1 -> y/1
  x/1 -> Gain/1

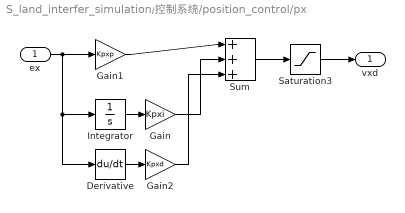
== system S_land_interfer_simulation/控制系统/position_control/px ==
  ex : Inport
  Derivative : Derivative
  Gain : Gain  Gain=Kpxi
  Gain1 : Gain  Gain=Kpxp
  Gain2 : Gain  Gain=Kpxd
  Integrator : Integrator
  Saturation3 : Saturate  UpperLimit=MAX_CONTROL_VELOCITY_XY  LowerLimit=-MAX_CONTROL_VELOCITY_XY
  Sum : Sum  Inputs=|+++
  vxd : Outport
  wires:
  ex/1 -> Derivative/1, Integrator/1, Gain1/1
  Saturation3/1 -> vxd/1
  Gain1/1 -> Sum/1
  Integrator/1 -> Gain/1
  Sum/1 -> Saturation3/1
  Gain/1 -> Sum/2
  Derivative/1 -> Gain2/1
  Gain2/1 -> Sum/3

== system S_land_interfer_simulation/控制系统/position_control/py ==
  ey : Inport
  Gain1 : Gain  Gain=Kpyp
  Saturation3 : Saturate  UpperLimit=MAX_CONTROL_VELOCITY_XY  LowerLimit=-MAX_CONTROL_VELOCITY_XY
  vyd : Outport
  wires:
  Gain1/1 -> Saturation3/1
  Saturation3/1 -> vyd/1
  ey/1 -> Gain1/1

== system S_land_interfer_simulation/控制系统/position_control/pz ==
  ez : Inport
  PID Controller : pid_lib/PID Controller  Controller=PID  Form=Parallel  TimeDomain=Continuous-time  UseExternalTs=off  SampleTime=-1  IntegratorMethod=Forward Euler  FilterMethod=Forward Euler  ControllerParametersSource=internal  P=Kpzp  I=Kpzi  D=Kpzd  UseFilter=on  N=100  TunerSelectOption=Transfer Function Based (PID Tuner App)  InitialConditionSource=internal  InitialConditionForIntegrator=0  InitialConditionForFilter=0  DifferentiatorICPrevScaledInput=0  ExternalReset=none  TrackingMode=off  Kt=1  LimitOutput=off  SatLimitsSource=internal  UpperSaturationLimit=inf  LowerSaturationLimit=-inf  LinearizeAsGain=on  AntiWindupMode=none  Kb=1  POutMin=[]  POutMax=[]  IOutMin=[]  IOutMax=[]  DOutMin=[]  DOutMax=[]  NOutMin=[]  NOutMax=[]  SumOutMin=[]  SumOutMax=[]  SaturationOutMin=[]  SaturationOutMax=[]  PParamMin=[]  PParamMax=[]  IParamMin=[]  IParamMax=[]  DParamMin=[]  DParamMax=[]  NParamMin=[]  NParamMax=[]  KbParamMin=[]  KbParamMax=[]  KtParamMin=[]  KtParamMax=[]  KbOutMin=[]  KbOutMax=[]  KtOutMin=[]  KtOutMax=[]  IntegratorOutMin=[]  IntegratorOutMax=[]  FilterOutMin=[]  FilterOutMax=[]  SumI1OutMin=[]  SumI1OutMax=[]  SumI2OutMin=[]  SumI2OutMax=[]  SumI3OutMin=[]  SumI3OutMax=[]  SumI4OutMin=[]  SumI4OutMax=[]  SumDOutMin=[]  SumDOutMax=[]  DifferentiatorOutMin=[]  DifferentiatorOutMax=[]  FilterDiffOutCoefMin=[]  FilterDiffOutCoefMax=[]  ReciprocalOutMin=[]  ReciprocalOutMax=[]  SumDenOutMin=[]  SumDenOutMax=[]  SumNumOutMin=[]  SumNumOutMax=[]  DivideOutMin=[]  DivideOutMax=[]  UdiffTsProdOutMin=[]  UdiffTsProdOutMax=[]  NTsProdOutMin=[]  NTsProdOutMax=[]  UintegralTsProdOutMin=[]  UintegralTsProdOutMax=[]  UngainTsProdOutMin=[]  UngainTsProdOutMax=[]  IntegratorContinuousStateAttributes=''  IntegratorStateMustResolveToSignalObject=off  IntegratorRTWStateStorageClass=Auto  FilterContinuousStateAttributes=''  FilterStateMustResolveToSignalObject=off  FilterRTWStateStorageClass=Auto  ParallelPVariant=InternalParameters  IdealPVariant=Disabled  IVariant=InternalParameters  DVariant=InternalParameters  IntegratorVariant=Continuous  SatVariant=Disabled  AWVariant=Passthrough  PCopyVariant=Disabled  TRVariant=Disabled  FdbkBlocksVariant=Forward  IdealPFdbkVariant=Disabled  SatFdbkVariant=Disabled  DerivativeFilterVariant=ContFilter  NVariant=InternalParameters  NCopyVariant=Disabled  FilterICVariant=InternalICsFilter  IntegratorICVariant=InternalICs  ExternalResetVariant=Disabled  TRSumVariant=Passthrough  SumFdbkVariant=Disabled  SumVariant=Sum_PID  TsampFilterVariant=InternalTs  TsampNgainVariant=Passthrough  TsampIntegralVariant=Passthrough  ExternalSaturationOutDataTypeStr=Inherit: Same as second input
  Saturation3 : Saturate  UpperLimit=MAX_CONTROL_VELOCITY_Z  LowerLimit=-MAX_CONTROL_VELOCITY_Z
  vzd : Outport
  wires:
  ez/1 -> PID Controller/1
  Saturation3/1 -> vzd/1
  PID Controller/1 -> Saturation3/1

== system S_land_interfer_simulation/控制系统/position_control/vy  ==
  x : Inport
  Derivative Gain : Gain  DisableCoverage=on  Gain=Kvyd
  Discrete Derivative : simulink/Discrete/Discrete Derivative  gainval=1.0  ICPrevScaledInput=0.0  OutMin=-5  OutMax=5  OutDataType=fixdt(1, 16)  OutScaling=2^-10  DoSatur=off
  Discrete-Time Integrator : DiscreteIntegrator  SampleTime=-1  LimitOutput=on  UpperSaturationLimit=Saturation_I_ah  LowerSaturationLimit=-Saturation_I_ah  ICPrevOutput=DiscIntNeverNeededParam  ICPrevScaledInput=DiscIntNeverNeededParam
  Gain : Gain  Gain=Kvyp
  Integral Gain : Gain  DisableCoverage=on  Gain=Kvyi
  Sum : Sum  Inputs=+++  OutMin=-5  OutMax=5
  y : Outport  InitialOutput=0
  wires:
  x/1 -> Gain/1, Integral Gain/1, Derivative Gain/1
  Integral Gain/1 -> Discrete-Time Integrator/1
  Derivative Gain/1 -> Discrete Derivative/1
  Gain/1 -> Sum/1
  Sum/1 -> y/1
  Discrete Derivative/1 -> Sum/3
  Discrete-Time Integrator/1 -> Sum/2

== system S_land_interfer_simulation/控制系统/position_control/vz  ==
  x : Inport
  Derivative Gain : Gain  DisableCoverage=on  Gain=Kvzd
  Discrete Derivative : simulink/Discrete/Discrete Derivative  gainval=1.0  ICPrevScaledInput=0.0  OutMin=[]  OutMax=[]  OutDataType=fixdt(1, 16)  OutScaling=2^-10  DoSatur=off
  Discrete-Time Integrator : DiscreteIntegrator  SampleTime=-1  LimitOutput=on  UpperSaturationLimit=Saturation_I_az  LowerSaturationLimit=-Saturation_I_az  ICPrevOutput=DiscIntNeverNeededParam  ICPrevScaledInput=DiscIntNeverNeededParam
  Gain : Gain  Gain=Kvzp
  Integral Gain : Gain  DisableCoverage=on  Gain=Kvzi
  Sum : Sum  Inputs=+++
  y : Outport  InitialOutput=0
  wires:
  Discrete-Time Integrator/1 -> Sum/2
  Discrete Derivative/1 -> Sum/3
  Sum/1 -> y/1
  Gain/1 -> Sum/1
  Derivative Gain/1 -> Discrete Derivative/1
  Integral Gain/1 -> Discrete-Time Integrator/1
  x/1 -> Derivative Gain/1, Integral Gain/1, Gain/1

== system S_land_interfer_simulation/四旋翼动力学模型 /刚体模型/刚体动力学模型/J*w ==
  p q r : Inport
  J : Inport  Port=2
  J*w : Product  Multiplication=Matrix(*)
  "J*w " : Outport
  wires:
  J*w/1 -> "J*w "/1
  J/1 -> J*w/1
  p q r/1 -> J*w/2

== matlab function S_land_interfer_simulation/控制系统/position_control/MATLAB Function ==
  data: eax input; eay input; psi input; phi output; theta output
function [phi,theta] = fcn(eax,eay,psi)
g=9.8;
phi = (-sin(psi)*eax + cos(psi)*eay)/g;
theta = (-cos(psi)*eax-sin(psi)*eay)/g;

== matlab function S_land_interfer_simulation/控制系统/pwm_out2 ==
  data: Roll input; M1 output; Pitch input; Yaw input; Thrust input; M2 output; M3 output; M4 output
function [M1, M2, M3, M4] = motor_mixer(Roll, Pitch, Yaw, Thrust)
%quadrotorX
%3     1
%  \ /
%  / \
%2     4

idle_PWM = 1000;
scale = 1000;

M1 = (Thrust - Roll + Pitch + Yaw) * scale + idle_PWM;
M2 = (Thrust + Roll - Pitch + Yaw) * scale + idle_PWM;
M3 = (Thrust + Roll + Pitch - Yaw) * scale + idle_PWM;
M4 = (Thrust - Roll - Pitch - Yaw) * scale + idle_PWM;

== matlab function S_land_interfer_simulation/四旋翼动力学模型 /刚体模型/刚体动力学模型/陀螺力矩 ==
  data: Jrp input; MotorRads input; pqr input; Ga output
function Ga = fcn(Jrp,MotorRads,pqr)
Ga=zeros(3,1);
Ga(1)=Jrp*pqr(2)*(-MotorRads(1)-MotorRads(2)+MotorRads(3)+MotorRads(4));
Ga(2)=Jrp*pqr(1)*( MotorRads(1)+MotorRads(2)-MotorRads(3)-MotorRads(4));

== matlab function S_land_interfer_simulation/四旋翼动力学模型 /刚体模型/计算旋转矩阵和欧拉角/四元数转欧拉角 ==
  data: q input; y output
function y = fcn(q)
Rbe = [q(1)*q(1) + q(2)*q(2) - q(3)*q(3) - q(4)*q(4), 2*(q(2)*q(3) - q(1)*q(4)), 2*(q(2)*q(4) + q(1)*q(3))
       2*(q(2)*q(3) + q(1)*q(4)), q(1)*q(1) - q(2)*q(2) + q(3)*q(3) - q(4)*q(4), 2*(q(3)*q(4) - q(1)*q(2))
       2*(q(2)*q(4) - q(1)*q(3)), 2*(q(3)*q(4) + q(1)*q(2)), q(1)*q(1) - q(2)*q(2) - q(3)*q(3) + q(4)*q(4)];
   
phi = atan2(Rbe(3,2),Rbe(3,3));
theta = asin(-Rbe(3,1));
psi = atan2(Rbe(2,1),Rbe(1,1));  
% phi = atan2(2*(q(1)*q(2)+q(3)*q(4)),(1-2*(q(2)*q(2)+q(3)*q(3))));
% theta = asin(2*(q(1)*q(3)-q(2)*q(4)));
% psi = atan2(2*(q(1)*q(4)+q(2)*q(3)),(1-2*(q(3)*q(3))+q(4)*q(4)));
y = [phi theta psi];

== matlab function S_land_interfer_simulation/四旋翼动力学模型 /刚体模型/计算旋转矩阵和欧拉角/基于四元数模型 ==
  data: pqr input; qdot output; q input
function qdot = fcn(pqr,q)

qdot=0.5*[0,-pqr(1),-pqr(2),-pqr(3);pqr(1),0,pqr(3),-pqr(2);pqr(2),-pqr(3),0,pqr(1);pqr(3),pqr(2),-pqr(1),0]*q;

== matlab function S_land_interfer_simulation/四旋翼动力学模型 /控制效率模型/Propeller Model ==
  data: w input; R input; Fb output; Fd output; Mb output; Cm input; Ct input; Vb input; Cd input
function [Fb,Fd,Mb] = fcn(w,R,Cm,Ct,Vb,Cd)
 %%叉字型
 %3  1
 %2  4
 M_rctcm = [-sin(pi/4)*R*Ct,sin(pi/4)*R*Ct,sin(pi/4)*R*Ct,-sin(pi/4)*R*Ct;
            sin(pi/4)*R*Ct,-sin(pi/4)*R*Ct,sin(pi/4)*R*Ct,-sin(pi/4)*R*Ct;
            Cm,Cm,-Cm,-Cm];
 Mb = M_rctcm*(w.^2);%式(6.24),力矩
 
 Fb = [0; 0; -sum(Ct*(w.^2))]; %(6.23),螺旋桨拉力
 Fd = -Cd*Vb.*abs(Vb)*0.5;%空气阻力
end
